simulink model "Bio_Digital_Twin"  (R2025b)
settings: Solver=VariableStepAuto  StartTime=0.0  StopTime=10.0  RelTol=1e-3
undefined symbols (not defined in the file): dspblkCoreblockFVToolHelper, gcbh
libraries: simulink x15, dspstat3 x4
(part 2 of 2)

== system Bio_Digital_Twin/Frugal_AI/4.5_Risk_Fusion_Decision_logic ==
  In1 : Inport  OutDataTypeStr=double
  SPO2_Mean : Inport  Port=2  OutDataTypeStr=double
  HR_Mean : Inport  Port=3  OutDataTypeStr=double
  In2 : Inport  Port=4  OutDataTypeStr=double
  Global_Health_State : Inport  Port=5  OutDataTypeStr=double
  Temp_Mean : Inport  Port=6  OutDataTypeStr=double
  In4 : Inport  Port=7  OutDataTypeStr=double
  HR_Flag : Inport  Port=8  OutDataTypeStr=double
  SPO2_Flag : Inport  Port=9  OutDataTypeStr=double
  TEMP_Flag : Inport  Port=10  OutDataTypeStr=double
  4.5.1_Risk_Signal_Normalizer : Subsystem
      settings: PortSchema="{\"entries\":[{\"content\":{\"sides\":[{\"content\":{},\"type\":\"ConnectorPlacement.EquallySpacedRectSide\",\"uuid\":\"8f35f634-c66e-422d-9c58-c61a4ee3cb54\"},{\"content\":{\"connectorIds\":[\"Out1\",\"Out2\",\"Out3\"],\"side\":\"RIGHT\"},\"type\":\"ConnectorPlacement.EquallySpacedRectSide\",\"uuid\":\"9f9283e6-4c64-451c-ad49-820c1276ee73\"},{\"content\":{\"side\":\"TOP\"},\"type\":\"ConnectorPlacement.EquallySpacedRectSide\",\"uuid\":\"18598fd6-31f1-4989-a958-abe44ef931de\"},{\"content\":{\"connectorIds\":[\"In1\",\"In2\",\"In3\"],\"side\":\"BOTTOM\"},\"type\":\"ConnectorPlacement.EquallySpacedRectSide\",\"uuid\":\"37672f05-fc1d-406b-b410-c6708a58aa07\"}]},\"type\":\"ConnectorPlacement.EquallySpacedConnector\",\"uuid\":\"a95a04c5-95c4-48ce-b08e-1a83caf92d36\"}],\"packageUris\":[\"http://schema.mathworks.com/mf0/Connector/R2020b\"],\"version\":\"1.0\"}"
  4.5.2_Physiological_Context_Moniter : Subsystem
      settings: PortSchema="{\"entries\":[{\"content\":{\"sides\":[{\"content\":{},\"type\":\"ConnectorPlacement.EquallySpacedRectSide\",\"uuid\":\"ba542400-0cd1-4e31-b99c-7003472743bf\"},{\"content\":{\"connectorIds\":[\"Out1\",\"Out2\",\"Out3\"],\"side\":\"RIGHT\"},\"type\":\"ConnectorPlacement.EquallySpacedRectSide\",\"uuid\":\"eb7b6bce-55bf-4921-bc52-6edeb25fab9e\"},{\"content\":{\"connectorIds\":[\"In1\",\"In2\",\"In3\"],\"side\":\"TOP\"},\"type\":\"ConnectorPlacement.EquallySpacedRectSide\",\"uuid\":\"71120ea0-ac95-49d2-9d4b-92656524cc31\"}]},\"type\":\"ConnectorPlacement.EquallySpacedConnector\",\"uuid\":\"9e07e074-34e6-4f09-a71b-3d251b7224e4\"}],\"packageUris\":[\"http://schema.mathworks.com/mf0/Connector/R2020b\"],\"version\":\"1.0\"}"
  4.5.3_Weighted_Risk_Fusion_Core : Subsystem
      settings: PortSchema="{\"entries\":[{\"content\":{\"sides\":[{\"content\":{\"connectorIds\":[\"In1\",\"In2\",\"In3\"]},\"type\":\"ConnectorPlacement.EquallySpacedRectSide\",\"uuid\":\"8f35f634-c66e-422d-9c58-c61a4ee3cb54\"},{\"content\":{\"connectorIds\":[\"Out1\"],\"side\":\"RIGHT\"},\"type\":\"ConnectorPlacement.EquallySpacedRectSide\",\"uuid\":\"9f9283e6-4c64-451c-ad49-820c1276ee73\"},{\"content\":{\"connectorIds\":[\"In4\",\"In5\",\"In6\"],\"side\":\"TOP\"},\"type\":\"ConnectorPlacement.EquallySpacedRectSide\",\"uuid\":\"18598fd6-31f1-4989-a958-abe44ef931de\"}]},\"type\":\"ConnectorPlacement.EquallySpacedConnector\",\"uuid\":\"a95a04c5-95c4-48ce-b08e-1a83caf92d36\"}],\"packageUris\":[\"http://schema.mathworks.com/mf0/Connector/R2020b\"],\"version\":\"1.0\"}"
  4.5.4_Discrete_Override_Logic : Subsystem
      settings: PortSchema="{\"entries\":[{\"content\":{\"sides\":[{\"content\":{},\"type\":\"ConnectorPlacement.EquallySpacedRectSide\",\"uuid\":\"ba542400-0cd1-4e31-b99c-7003472743bf\"},{\"content\":{\"connectorIds\":[\"Out1\",\"Out2\"],\"side\":\"RIGHT\"},\"type\":\"ConnectorPlacement.EquallySpacedRectSide\",\"uuid\":\"eb7b6bce-55bf-4921-bc52-6edeb25fab9e\"},{\"content\":{\"connectorIds\":[\"In1\"],\"side\":\"TOP\"},\"type\":\"ConnectorPlacement.EquallySpacedRectSide\",\"uuid\":\"71120ea0-ac95-49d2-9d4b-92656524cc31\"},{\"content\":{\"connectorIds\":[\"In2\",\"In3\",\"In4\",\"In5\"],\"side\":\"BOTTOM\"},\"type\":\"ConnectorPlacement.EquallySpacedRectSide\",\"uuid\":\"ed423af9-15f8-4a33-aaec-371b081b1cbe\"}]},\"type\":\"ConnectorPlacement.EquallySpacedConnector\",\"uuid\":\"9e07e074-34e6-4f09-a71b-3d251b7224e4\"}],\"packageUris\":[\"http://schema.mathworks.com/mf0/Connector/R2020b\"],\"version\":\"1.0\"}"
  4.5.5_Final_Risk_Selecter&Decision_Output : Subsystem
      settings: PortSchema="{\"entries\":[{\"content\":{\"sides\":[{\"content\":{\"connectorIds\":[\"In1\",\"In2\"]},\"type\":\"ConnectorPlacement.EquallySpacedRectSide\",\"uuid\":\"1398e62b-675a-459d-b341-3a2d58b0042e\"},{\"content\":{\"connectorIds\":[\"Out1\",\"Out2\",\"Out3\",\"Out4\"],\"side\":\"RIGHT\"},\"type\":\"ConnectorPlacement.EquallySpacedRectSide\",\"uuid\":\"49b971ab-5b3e-431b-b022-6e647649d68a\"},{\"content\":{\"connectorIds\":[\"In3\",\"Out5\"],\"side\":\"TOP\"},\"type\":\"ConnectorPlacement.EquallySpacedRectSide\",\"uuid\":\"481e4b75-ca94-4b8e-ac5a-54646a036782\"}]},\"type\":\"ConnectorPlacement.EquallySpacedConnector\",\"uuid\":\"3a2d46a4-3de7-4d3b-b474-f54ea7c5581f\"}],\"packageUris\":[\"http://schema.mathworks.com/mf0/Connector/R2020b\"],\"version\":\"1.0\"}"
  Scope : Scope
      settings: DataLoggingVariableName=ScopeData76  DataLoggingSaveFormat=Array
  Scope1 : Scope
      settings: DataLoggingVariableName=ScopeData77  DataLoggingSaveFormat=Array
  Risk_Level : Outport
  Global_Risk_Index : Outport  Port=2
  Over_Ride_Flag : Outport  Port=3
  wires:
  In1/1 -> 4.5.1_Risk_Signal_Normalizer/1(HR_Risk_Score)
  In2/1 -> 4.5.1_Risk_Signal_Normalizer/3(SPO2_Risk_Score)
  In4/1 -> 4.5.1_Risk_Signal_Normalizer/2(TEMP_Risk_Score)
  HR_Mean/1 -> 4.5.2_Physiological_Context_Moniter/1(HR_Mean)
  SPO2_Mean/1 -> 4.5.2_Physiological_Context_Moniter/2(SPO2_Mean)
  Temp_Mean/1 -> 4.5.2_Physiological_Context_Moniter/3(Temp_Mean)
  4.5.2_Physiological_Context_Moniter/1(HR_Context_Risk) -> 4.5.3_Weighted_Risk_Fusion_Core/6(HR_Context_Risk)
  4.5.2_Physiological_Context_Moniter/2(TEMP_Context_Risk) -> 4.5.3_Weighted_Risk_Fusion_Core/3(TEMP_Context_Risk)
  4.5.2_Physiological_Context_Moniter/3(SPO2_Context_Risk) -> 4.5.3_Weighted_Risk_Fusion_Core/1(SPO2_Context_Risk)
  Global_Health_State/1 -> 4.5.4_Discrete_Override_Logic/2(Global_Health_State)
  4.5.3_Weighted_Risk_Fusion_Core/1(Global_Risk_Index) -> 4.5.5_Final_Risk_Selecter&Decision_Output/3(Global_Risk_Index), 4.5.4_Discrete_Override_Logic/1(Global_Risk_Index)
  HR_Flag/1 -> 4.5.4_Discrete_Override_Logic/3(HR_Flag)
  SPO2_Flag/1 -> 4.5.4_Discrete_Override_Logic/5(SPO2_Flag)
  TEMP_Flag/1 -> 4.5.4_Discrete_Override_Logic/4(TEMP_Flag)
  4.5.1_Risk_Signal_Normalizer/1(HR_Risk_Norm) -> 4.5.3_Weighted_Risk_Fusion_Core/5(HR_Risk_Norm)
  4.5.1_Risk_Signal_Normalizer/2(SPO2_Risk_Norm) -> 4.5.3_Weighted_Risk_Fusion_Core/4(SPO2_Risk_Norm)
  4.5.1_Risk_Signal_Normalizer/3(TEMP_Risk_Norm) -> 4.5.3_Weighted_Risk_Fusion_Core/2(TEMP_Risk_Norm)
  4.5.4_Discrete_Override_Logic/1(Override_level) -> 4.5.5_Final_Risk_Selecter&Decision_Output/2(Override_level)
  4.5.4_Discrete_Override_Logic/2(Out1) -> 4.5.5_Final_Risk_Selecter&Decision_Output/1(Override_Flag)
  4.5.5_Final_Risk_Selecter&Decision_Output/1(Out1) -> Scope/1
  4.5.5_Final_Risk_Selecter&Decision_Output/2(Out2) -> Scope1/1
  4.5.5_Final_Risk_Selecter&Decision_Output/5(Out3) -> Global_Risk_Index/1
  4.5.5_Final_Risk_Selecter&Decision_Output/3(Out4) -> Risk_Level/1
  4.5.5_Final_Risk_Selecter&Decision_Output/4(Out5) -> Over_Ride_Flag/1

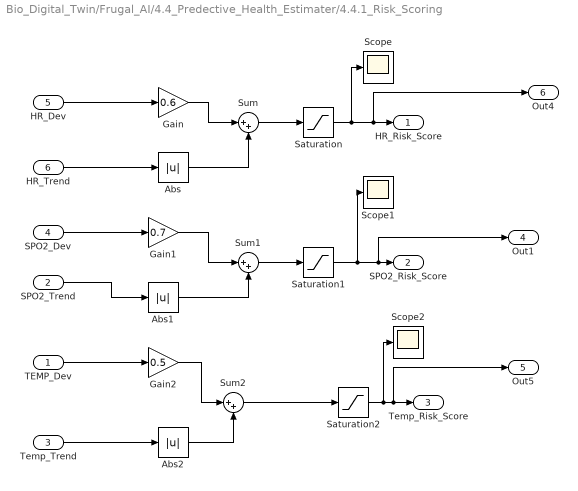
== system Bio_Digital_Twin/Frugal_AI/4.4_Predective_Health_Estimater/4.4.1_Risk_Scoring ==
  TEMP_Dev : Inport
  SPO2_Trend : Inport  Port=2
  Temp_Trend : Inport  Port=3
  SPO2_Dev : Inport  Port=4
  HR_Dev : Inport  Port=5  OutDataTypeStr=double
  HR_Trend : Inport  Port=6
  Abs : Abs  ZeroCross=off  OutDataTypeStr=double  SaturateOnIntegerOverflow=off
  Abs1 : Abs  ZeroCross=off  SaturateOnIntegerOverflow=off
  Abs2 : Abs  ZeroCross=off  SaturateOnIntegerOverflow=off
  Gain : Gain  Gain=0.6
  Gain1 : Gain  Gain=0.7
  Gain2 : Gain  Gain=0.5
  Saturation : Saturate  UpperLimit=1  LowerLimit=0  ZeroCross=off
  Saturation1 : Saturate  UpperLimit=1  LowerLimit=0  ZeroCross=off
  Saturation2 : Saturate  UpperLimit=1  LowerLimit=0  ZeroCross=off
  Scope : Scope
      settings: DataLoggingVariableName=ScopeData38  DataLoggingSaveFormat=Array
  Scope1 : Scope
      settings: ActiveDisplayYMinimum=-0.029651653403424238  ActiveDisplayYMaximum=1.5657002997215752  DataLoggingVariableName=ScopeData39  DataLoggingSaveFormat=Array
  Scope2 : Scope
      settings: DataLoggingVariableName=ScopeData40  DataLoggingSaveFormat=Array
  Sum : Sum  Inputs=|++
  Sum1 : Sum  Inputs=|++
  Sum2 : Sum  Inputs=|++
  HR_Risk_Score : Outport  VectorParamsAs1DForOutWhenUnconnected=off
  SPO2_Risk_Score : Outport  Port=2  VectorParamsAs1DForOutWhenUnconnected=off
  Temp_Risk_Score : Outport  Port=3  VectorParamsAs1DForOutWhenUnconnected=off
  Out1 : Outport  Port=4
  Out5 : Outport  Port=5
  Out4 : Outport  Port=6
  wires:
  HR_Trend/1 -> Abs/1
  HR_Dev/1 -> Gain/1
  Gain/1 -> Sum/1
  Abs/1 -> Sum/2
  Sum/1 -> Saturation/1
  Saturation/1 -> Scope/1, Out4/1, HR_Risk_Score/1
  SPO2_Dev/1 -> Gain1/1
  SPO2_Trend/1 -> Abs1/1
  Gain1/1 -> Sum1/1
  Abs1/1 -> Sum1/2
  Sum1/1 -> Saturation1/1
  Saturation1/1 -> Scope1/1, Out1/1, SPO2_Risk_Score/1
  TEMP_Dev/1 -> Gain2/1
  Temp_Trend/1 -> Abs2/1
  Gain2/1 -> Sum2/1
  Abs2/1 -> Sum2/2
  Sum2/1 -> Saturation2/1
  Saturation2/1 -> Scope2/1, Out5/1, Temp_Risk_Score/1

== system Bio_Digital_Twin/Frugal_AI/4.4_Predective_Health_Estimater/4.4.2_Trend_Penetration ==
  HR_Trend : Inport
  SPO2_Trend : Inport  Port=2
  Temp_Trend : Inport  Port=3
  Abs : Abs  ZeroCross=off  SaturateOnIntegerOverflow=off
  Abs1 : Abs  ZeroCross=off  SaturateOnIntegerOverflow=off
  Abs2 : Abs  ZeroCross=off  SaturateOnIntegerOverflow=off
  Gain : Gain  Gain=0.3
  Gain1 : Gain  Gain=0.6
  Gain2 : Gain  Gain=1.2
  Saturation : Saturate  UpperLimit=0.3  LowerLimit=0  ZeroCross=off
  Saturation1 : Saturate  UpperLimit=0.20  LowerLimit=0  ZeroCross=off
  Saturation2 : Saturate  UpperLimit=0.25  LowerLimit=0  ZeroCross=off
  Scope : Scope
      settings: ActiveDisplayYMinimum=-0.037499999999999992  ActiveDisplayYMaximum=0.33749999999999997  DataLoggingVariableName=ScopeData41  DataLoggingSaveFormat=Array
  Scope1 : Scope
      settings: ActiveDisplayYMinimum=-0.024999999999999994  ActiveDisplayYMaximum=0.225  DataLoggingVariableName=ScopeData42  DataLoggingSaveFormat=Array
  Scope2 : Scope
      settings: ActiveDisplayYMinimum=-0.031249999999999993  ActiveDisplayYMaximum=0.28125  DataLoggingVariableName=ScopeData43  DataLoggingSaveFormat=Array
  HR_Trend_Penalty : Outport
  SPO2_Trend_Penality : Outport  Port=2
  TEMP_Penality : Outport  Port=3
  wires:
  HR_Trend/1 -> Abs/1
  Saturation/1 -> Scope/1, HR_Trend_Penalty/1
  Gain/1 -> Saturation/1
  Abs/1 -> Gain/1
  SPO2_Trend/1 -> Abs1/1
  Temp_Trend/1 -> Abs2/1
  Abs2/1 -> Gain2/1
  Gain2/1 -> Saturation2/1
  Saturation2/1 -> Scope2/1, TEMP_Penality/1
  Abs1/1 -> Gain1/1
  Gain1/1 -> Saturation1/1
  Saturation1/1 -> Scope1/1, SPO2_Trend_Penality/1

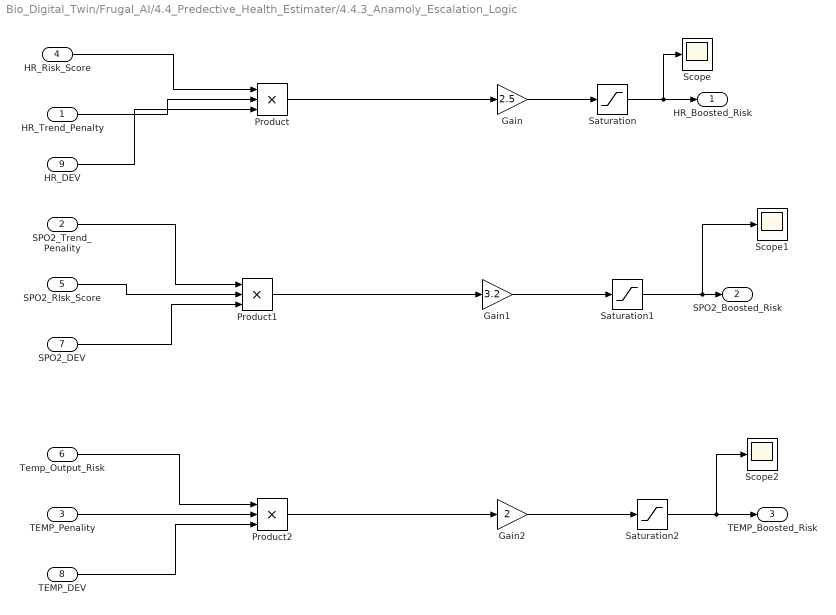
== system Bio_Digital_Twin/Frugal_AI/4.4_Predective_Health_Estimater/4.4.3_Anamoly_Escalation_Logic ==
  HR_Trend_Penalty : Inport
  SPO2_Trend_Penality : Inport  Port=2
  TEMP_Penality : Inport  Port=3
  HR_Risk_Score : Inport  Port=4
  SPO2_RIsk_Score : Inport  Port=5
  Temp_Output_Risk : Inport  Port=6
  SPO2_DEV : Inport  Port=7
  TEMP_DEV : Inport  Port=8
  HR_DEV : Inport  Port=9
  Gain : Gain  Gain=2.5
  Gain1 : Gain  Gain=3.2
  Gain2 : Gain  Gain=2
  Product : Product  Inputs=3
  Product1 : Product  Inputs=3
  Product2 : Product  Inputs=3
  Saturation : Saturate  UpperLimit=1  LowerLimit=0  ZeroCross=off
  Saturation1 : Saturate  UpperLimit=1  LowerLimit=0  ZeroCross=off
  Saturation2 : Saturate  UpperLimit=1  LowerLimit=0  ZeroCross=off
  Scope : Scope
      settings: ActiveDisplayYMinimum=-0.076388475038902851  ActiveDisplayYMaximum=0.68749627535012581  DataLoggingVariableName=ScopeData44  DataLoggingSaveFormat=Array
  Scope1 : Scope
      settings: ActiveDisplayYMinimum=-0.067702104531752558  ActiveDisplayYMaximum=0.60931894078577309  DataLoggingVariableName=ScopeData45  DataLoggingSaveFormat=Array
  Scope2 : Scope
      settings: ActiveDisplayYMinimum=-0.0094894903527777043  ActiveDisplayYMaximum=0.085405413174999362  DataLoggingVariableName=ScopeData46  DataLoggingSaveFormat=Array
  HR_Boosted_Risk : Outport  VectorParamsAs1DForOutWhenUnconnected=off
  SPO2_Boosted_Risk : Outport  Port=2
  TEMP_Boosted_Risk : Outport  Port=3
  wires:
  HR_Risk_Score/1 -> Product/1
  HR_Trend_Penalty/1 -> Product/2
  HR_DEV/1 -> Product/3
  SPO2_Trend_Penality/1 -> Product1/1
  SPO2_RIsk_Score/1 -> Product1/2
  SPO2_DEV/1 -> Product1/3
  Temp_Output_Risk/1 -> Product2/1
  TEMP_Penality/1 -> Product2/2
  TEMP_DEV/1 -> Product2/3
  Product/1 -> Gain/1
  Gain/1 -> Saturation/1
  Saturation/1 -> Scope/1, HR_Boosted_Risk/1
  Gain2/1 -> Saturation2/1
  Gain1/1 -> Saturation1/1
  Saturation1/1 -> Scope1/1, SPO2_Boosted_Risk/1
  Saturation2/1 -> Scope2/1, TEMP_Boosted_Risk/1
  Product1/1 -> Gain1/1
  Product2/1 -> Gain2/1

== system Bio_Digital_Twin/Frugal_AI/4.4_Predective_Health_Estimater/4.4.4_Vital_Fusion_Engine ==
  SPO2_Trend_Penality : Inport
  TEMP_Boosted_Risk : Inport  Port=2
  HR_Boosted_Risk : Inport  Port=3
  TEMP_Trend_Penality : Inport  Port=4
  TEMP_Flag : Inport  Port=5
  HR_Trend_Penalty : Inport  Port=6
  HR_Flag : Inport  Port=7
  SPO2_Flag : Inport  Port=8
  SPO2_Boosted_Risk : Inport  Port=9
  4.4.4.1_Weighted_Risk_Aggregator : Subsystem
      settings: PortSchema="{\"entries\":[{\"content\":{\"sides\":[{\"content\":{},\"type\":\"ConnectorPlacement.EquallySpacedRectSide\",\"uuid\":\"737bb885-e7c9-4573-85e5-b83dda6485f1\"},{\"content\":{\"connectorIds\":[\"Out1\"],\"side\":\"RIGHT\"},\"type\":\"ConnectorPlacement.EquallySpacedRectSide\",\"uuid\":\"740a03a9-133d-4f41-bb19-7b5e8b3a8d7e\"},{\"content\":{\"connectorIds\":[\"In1\"],\"side\":\"TOP\"},\"type\":\"ConnectorPlacement.EquallySpacedRectSide\",\"uuid\":\"4008c6be-6fbc-4f8a-ab91-2e671a35a61f\"},{\"content\":{\"connectorIds\":[\"In2\",\"In3\"],\"side\":\"BOTTOM\"},\"type\":\"ConnectorPlacement.EquallySpacedRectSide\",\"uuid\":\"541123af-325e-4018-abd6-217c806ff677\"}]},\"type\":\"ConnectorPlacement.EquallySpacedConnector\",\"uuid\":\"4bffb07e-74c2-4f1f-82f1-4306adc281b9\"}],\"packageUris\":[\"http://schema.mathworks.com/mf0/Connector/R2020b\"],\"version\":\"1.0\"}"
  4.4.4.2_Trend_Reinforcement_Logic : Subsystem
      settings: PortSchema="{\"entries\":[{\"content\":{\"sides\":[{\"content\":{},\"type\":\"ConnectorPlacement.EquallySpacedRectSide\",\"uuid\":\"25541af2-9525-4f8c-abbb-22df26048cee\"},{\"content\":{\"connectorIds\":[\"Out1\"],\"side\":\"RIGHT\"},\"type\":\"ConnectorPlacement.EquallySpacedRectSide\",\"uuid\":\"1363b628-3ee9-451f-9ff9-7a32b3bff014\"},{\"content\":{\"side\":\"TOP\"},\"type\":\"ConnectorPlacement.EquallySpacedRectSide\",\"uuid\":\"085c579b-f7a8-4980-bc39-19f414c4d171\"},{\"content\":{\"connectorIds\":[\"In1\",\"In2\",\"In3\"],\"side\":\"BOTTOM\"},\"type\":\"ConnectorPlacement.EquallySpacedRectSide\",\"uuid\":\"8648316c-16bf-41e8-ae35-abe9e87cf577\"}]},\"type\":\"ConnectorPlacement.EquallySpacedConnector\",\"uuid\":\"fb659e6d-00b5-4060-933b-4a03338751c4\"}],\"packageUris\":[\"http://schema.mathworks.com/mf0/Connector/R2020b\"],\"version\":\"1.0\"}"
  4.4.4.3_Flag_Confidence_Gate : Subsystem
      settings: PortSchema="{\"entries\":[{\"content\":{\"sides\":[{\"content\":{},\"type\":\"ConnectorPlacement.EquallySpacedRectSide\",\"uuid\":\"25541af2-9525-4f8c-abbb-22df26048cee\"},{\"content\":{\"connectorIds\":[\"Out1\"],\"side\":\"RIGHT\"},\"type\":\"ConnectorPlacement.EquallySpacedRectSide\",\"uuid\":\"1363b628-3ee9-451f-9ff9-7a32b3bff014\"},{\"content\":{\"connectorIds\":[\"In1\"],\"side\":\"TOP\"},\"type\":\"ConnectorPlacement.EquallySpacedRectSide\",\"uuid\":\"085c579b-f7a8-4980-bc39-19f414c4d171\"},{\"content\":{\"connectorIds\":[\"In2\",\"In3\",\"In4\"],\"side\":\"BOTTOM\"},\"type\":\"ConnectorPlacement.EquallySpacedRectSide\",\"uuid\":\"37001957-af6f-4dd2-a4d8-c32bc34d5802\"}]},\"type\":\"ConnectorPlacement.EquallySpacedConnector\",\"uuid\":\"fb659e6d-00b5-4060-933b-4a03338751c4\"}],\"packageUris\":[\"http://schema.mathworks.com/mf0/Connector/R2020b\"],\"version\":\"1.0\"}"
  4.4.4.4_Final_risk_Normalizer : Subsystem
  4.4.4.5_Decision&Drug_Trigger_Logic : Subsystem
      settings: PortSchema="{\"entries\":[{\"content\":{\"sides\":[{\"content\":{},\"type\":\"ConnectorPlacement.EquallySpacedRectSide\",\"uuid\":\"737bb885-e7c9-4573-85e5-b83dda6485f1\"},{\"content\":{\"connectorIds\":[\"Out1\"],\"side\":\"RIGHT\"},\"type\":\"ConnectorPlacement.EquallySpacedRectSide\",\"uuid\":\"740a03a9-133d-4f41-bb19-7b5e8b3a8d7e\"},{\"content\":{\"connectorIds\":[\"In1\"],\"side\":\"TOP\"},\"type\":\"ConnectorPlacement.EquallySpacedRectSide\",\"uuid\":\"4008c6be-6fbc-4f8a-ab91-2e671a35a61f\"}]},\"type\":\"ConnectorPlacement.EquallySpacedConnector\",\"uuid\":\"4bffb07e-74c2-4f1f-82f1-4306adc281b9\"}],\"packageUris\":[\"http://schema.mathworks.com/mf0/Connector/R2020b\"],\"version\":\"1.0\"}"
  wires:
  HR_Boosted_Risk/1 -> 4.4.4.1_Weighted_Risk_Aggregator/3(HR_Boosted_Risk)
  SPO2_Boosted_Risk/1 -> 4.4.4.1_Weighted_Risk_Aggregator/2(SPO2_Boosted_Risk)
  TEMP_Boosted_Risk/1 -> 4.4.4.1_Weighted_Risk_Aggregator/1(TEMP_Boosted_Risk)
  SPO2_Trend_Penality/1 -> 4.4.4.2_Trend_Reinforcement_Logic/1(SPO2_Trend_Penality)
  HR_Trend_Penalty/1 -> 4.4.4.2_Trend_Reinforcement_Logic/2(HR_Trend_Penalty)
  TEMP_Trend_Penality/1 -> 4.4.4.2_Trend_Reinforcement_Logic/3(TEMP_Trend_Penality)
  HR_Flag/1 -> 4.4.4.3_Flag_Confidence_Gate/2(HR_Flag)
  SPO2_Flag/1 -> 4.4.4.3_Flag_Confidence_Gate/4(SPO2_Flag)
  TEMP_Flag/1 -> 4.4.4.3_Flag_Confidence_Gate/3(TEMP_Flag)
  4.4.4.2_Trend_Reinforcement_Logic/1(Trend_Factor) -> 4.4.4.4_Final_risk_Normalizer/3(Trend_Factor), 4.4.4.3_Flag_Confidence_Gate/1(Trend_Factor)
  4.4.4.1_Weighted_Risk_Aggregator/1(R_Weighted) -> 4.4.4.4_Final_risk_Normalizer/1(R_Weighted)
  4.4.4.3_Flag_Confidence_Gate/1(Risk_Validated) -> 4.4.4.4_Final_risk_Normalizer/2(Risk_Validated)
  4.4.4.4_Final_risk_Normalizer/1(Vital_Risk_Score) -> 4.4.4.5_Decision&Drug_Trigger_Logic/1(Vital_Risk_Score)

== system Bio_Digital_Twin/Frugal_AI/4.4_Predective_Health_Estimater/4.4.5_Health_State_Encoder ==
  HR_Risk_Score : Inport  OutDataTypeStr=double
  SPO2_RIsk_Score : Inport  Port=2  OutDataTypeStr=double
  Temp_Risk_Output : Inport  Port=3  OutDataTypeStr=double
  TEMP_Flag : Inport  Port=4  OutDataTypeStr=double
  HR_Flag : Inport  Port=5
  SPO2_Flag : Inport  Port=6  OutDataTypeStr=double
  4.4.5.1_Vital_Severity_Normalizer : Subsystem
      settings: PortSchema="{\"entries\":[{\"content\":{\"sides\":[{\"content\":{\"connectorIds\":[\"In1\"]},\"type\":\"ConnectorPlacement.EquallySpacedRectSide\",\"uuid\":\"25541af2-9525-4f8c-abbb-22df26048cee\"},{\"content\":{\"connectorIds\":[\"In6\",\"Out1\",\"Out2\",\"Out3\"],\"side\":\"RIGHT\"},\"type\":\"ConnectorPlacement.EquallySpacedRectSide\",\"uuid\":\"1363b628-3ee9-451f-9ff9-7a32b3bff014\"},{\"content\":{\"side\":\"TOP\"},\"type\":\"ConnectorPlacement.EquallySpacedRectSide\",\"uuid\":\"085c579b-f7a8-4980-bc39-19f414c4d171\"},{\"content\":{\"connectorIds\":[\"In2\",\"In3\",\"In4\",\"In5\"],\"side\":\"BOTTOM\"},\"type\":\"ConnectorPlacement.EquallySpacedRectSide\",\"uuid\":\"3b4b4325-d39e-4c80-9f50-c26047788f8b\"}]},\"type\":\"ConnectorPlacement.EquallySpacedConnector\",\"uuid\":\"fb659e6d-00b5-4060-933b-4a03338751c4\"}],\"packageUris\":[\"http://schema.mathworks.com/mf0/Connector/R2020b\"],\"version\":\"1.0\"}"
  4.4.5.2_Health_Vector_Builder : Subsystem
  4.4.5.3_Weighted_Health_Index_generator : Subsystem
  4.4.5.4_Discrete_Health_State_Classifier : Subsystem
  4.4.5.5_Final_Decision : Subsystem
      settings: PortSchema="{\"entries\":[{\"content\":{\"sides\":[{\"content\":{\"connectorIds\":[\"In1\"]},\"type\":\"ConnectorPlacement.EquallySpacedRectSide\",\"uuid\":\"25541af2-9525-4f8c-abbb-22df26048cee\"},{\"content\":{\"connectorIds\":[\"Out1\"],\"side\":\"RIGHT\"},\"type\":\"ConnectorPlacement.EquallySpacedRectSide\",\"uuid\":\"1363b628-3ee9-451f-9ff9-7a32b3bff014\"},{\"content\":{\"connectorIds\":[\"In2\",\"In3\"],\"side\":\"TOP\"},\"type\":\"ConnectorPlacement.EquallySpacedRectSide\",\"uuid\":\"085c579b-f7a8-4980-bc39-19f414c4d171\"},{\"content\":{\"connectorIds\":[\"In4\"],\"side\":\"BOTTOM\"},\"type\":\"ConnectorPlacement.EquallySpacedRectSide\",\"uuid\":\"6701486d-dcdb-4b0d-ba3b-9fb711ea3ea4\"}]},\"type\":\"ConnectorPlacement.EquallySpacedConnector\",\"uuid\":\"fb659e6d-00b5-4060-933b-4a03338751c4\"}],\"packageUris\":[\"http://schema.mathworks.com/mf0/Connector/R2020b\"],\"version\":\"1.0\"}"
  Global_Health_State : Outport  OutDataTypeStr=double  VectorParamsAs1DForOutWhenUnconnected=off
  wires:
  TEMP_Flag/1 -> 4.4.5.1_Vital_Severity_Normalizer/1(TEMP_Flag)
  SPO2_Flag/1 -> 4.4.5.1_Vital_Severity_Normalizer/5(SPO2_Flag)
  HR_Flag/1 -> 4.4.5.1_Vital_Severity_Normalizer/6(HR_Flag)
  4.4.5.1_Vital_Severity_Normalizer/1(HR_Severity) -> 4.4.5.2_Health_Vector_Builder/1(HR_Severity)
  4.4.5.1_Vital_Severity_Normalizer/2(SPO2_Severity) -> 4.4.5.2_Health_Vector_Builder/2(SPO2_Severity)
  4.4.5.1_Vital_Severity_Normalizer/3(TEMP_Severity) -> 4.4.5.2_Health_Vector_Builder/3(TEMP_Severity)
  4.4.5.2_Health_Vector_Builder/1(Health_Vector) -> 4.4.5.3_Weighted_Health_Index_generator/1(Health_Vector)
  4.4.5.2_Health_Vector_Builder/2(Out1) -> 4.4.5.4_Discrete_Health_State_Classifier/1(HR_Severity)
  4.4.5.2_Health_Vector_Builder/3(Out2) -> 4.4.5.4_Discrete_Health_State_Classifier/2(SPO2_Severity)
  4.4.5.4_Discrete_Health_State_Classifier/1(HR_Health_State) -> 4.4.5.5_Final_Decision/2(HR_Health_State)
  4.4.5.4_Discrete_Health_State_Classifier/2(SPO2_Health_state) -> 4.4.5.5_Final_Decision/3(SPO2_Health_state)
  4.4.5.4_Discrete_Health_State_Classifier/3(TEMP_Health_State) -> 4.4.5.5_Final_Decision/4(TEMP_Health_State)
  4.4.5.2_Health_Vector_Builder/4(Out3) -> 4.4.5.4_Discrete_Health_State_Classifier/3(TEMP_Severity)
  HR_Risk_Score/1 -> 4.4.5.1_Vital_Severity_Normalizer/2(HR_Risk_Score)
  SPO2_RIsk_Score/1 -> 4.4.5.1_Vital_Severity_Normalizer/4(SPO2_RIsk_Score)
  Temp_Risk_Output/1 -> 4.4.5.1_Vital_Severity_Normalizer/3(Temp_Risk_Output)
  4.4.5.3_Weighted_Health_Index_generator/1(Health_Index) -> 4.4.5.5_Final_Decision/1(Health_Index)
  4.4.5.5_Final_Decision/1(Global_Health_State) -> Global_Health_State/1

== system Bio_Digital_Twin/Frugal_AI/4.5_Risk_Fusion_Decision_logic/4.5.1_Risk_Signal_Normalizer ==
  HR_Risk_Score : Inport  OutDataTypeStr=double
  TEMP_Risk_Score : Inport  Port=2  OutDataTypeStr=double
  SPO2_Risk_Score : Inport  Port=3  OutDataTypeStr=double
  Saturation : Saturate  UpperLimit=1  LowerLimit=0  ZeroCross=off  OutDataTypeStr=double
  Saturation1 : Saturate  UpperLimit=1  LowerLimit=0  ZeroCross=off  OutDataTypeStr=double
  Saturation2 : Saturate  UpperLimit=1  LowerLimit=0  ZeroCross=off  OutDataTypeStr=double
  Scope : Scope
      settings: DataLoggingVariableName=ScopeData64  DataLoggingSaveFormat=Array
  Scope1 : Scope
      settings: DataLoggingVariableName=ScopeData65  DataLoggingSaveFormat=Array
  Scope2 : Scope
      settings: DataLoggingVariableName=ScopeData66  DataLoggingSaveFormat=Array
  HR_Risk_Norm : Outport  OutDataTypeStr=double
  SPO2_Risk_Norm : Outport  Port=2  OutDataTypeStr=double
  TEMP_Risk_Norm : Outport  Port=3  OutDataTypeStr=double
  wires:
  HR_Risk_Score/1 -> Saturation/1
  Saturation/1 -> Scope/1, HR_Risk_Norm/1
  SPO2_Risk_Score/1 -> Saturation2/1
  TEMP_Risk_Score/1 -> Saturation1/1
  Saturation2/1 -> Scope2/1, SPO2_Risk_Norm/1
  Saturation1/1 -> TEMP_Risk_Norm/1, Scope1/1

== system Bio_Digital_Twin/Frugal_AI/4.5_Risk_Fusion_Decision_logic/4.5.2_Physiological_Context_Moniter ==
  HR_Mean : Inport  OutDataTypeStr=double
  SPO2_Mean : Inport  Port=2  OutDataTypeStr=double
  Temp_Mean : Inport  Port=3  OutDataTypeStr=double
  Gain : Gain  Gain=1/100  OutDataTypeStr=double
  Gain1 : Gain  Gain=1/100  OutDataTypeStr=double
  Gain2 : Gain  Gain=1/50  OutDataTypeStr=double
  Scope : Scope
      settings: DataLoggingVariableName=ScopeData68  DataLoggingSaveFormat=Array
  Scope1 : Scope
      settings: DataLoggingVariableName=ScopeData69  DataLoggingSaveFormat=Array
  Scope2 : Scope
      settings: DataLoggingVariableName=ScopeData70  DataLoggingSaveFormat=Array
  HR_Context_Risk : Outport  OutDataTypeStr=double
  TEMP_Context_Risk : Outport  Port=2  OutDataTypeStr=double
  SPO2_Context_Risk : Outport  Port=3  OutDataTypeStr=double
  wires:
  HR_Mean/1 -> Gain/1
  Temp_Mean/1 -> Gain2/1
  SPO2_Mean/1 -> Gain1/1
  Gain/1 -> Scope/1, HR_Context_Risk/1
  Gain2/1 -> Scope2/1, TEMP_Context_Risk/1
  Gain1/1 -> Scope1/1, SPO2_Context_Risk/1

== system Bio_Digital_Twin/Frugal_AI/4.5_Risk_Fusion_Decision_logic/4.5.3_Weighted_Risk_Fusion_Core ==
  SPO2_Context_Risk : Inport  OutDataTypeStr=double
  TEMP_Risk_Norm : Inport  Port=2  OutDataTypeStr=double
  TEMP_Context_Risk : Inport  Port=3  OutDataTypeStr=double
  SPO2_Risk_Norm : Inport  Port=4  OutDataTypeStr=double
  HR_Risk_Norm : Inport  Port=5  OutDataTypeStr=double
  HR_Context_Risk : Inport  Port=6  OutDataTypeStr=double
  Gain : Gain  Gain=0.4  OutDataTypeStr=double
  Gain1 : Gain  Gain=0.4  OutDataTypeStr=double
  Gain2 : Gain  Gain=0.4  OutDataTypeStr=double
  Gain3 : Gain  OutDataTypeStr=double
  Gain4 : Gain  OutDataTypeStr=double
  Gain5 : Gain  OutDataTypeStr=double
  Saturation : Saturate  UpperLimit=1  LowerLimit=0  ZeroCross=off  OutDataTypeStr=double
  Scope : Scope
      settings: DataLoggingVariableName=ScopeData71  DataLoggingSaveFormat=Array
  Sum : Sum  Inputs=|++++++  OutDataTypeStr=double
  Global_Risk_Index : Outport  OutDataTypeStr=double
  wires:
  HR_Context_Risk/1 -> Gain/1
  SPO2_Context_Risk/1 -> Gain2/1
  TEMP_Context_Risk/1 -> Gain1/1
  Gain/1 -> Sum/1
  Gain2/1 -> Sum/2
  Gain1/1 -> Sum/3
  Sum/1 -> Saturation/1
  Saturation/1 -> Scope/1, Global_Risk_Index/1
  SPO2_Risk_Norm/1 -> Gain3/1
  Gain3/1 -> Sum/4
  HR_Risk_Norm/1 -> Gain5/1
  Gain5/1 -> Sum/5
  Gain4/1 -> Sum/6
  TEMP_Risk_Norm/1 -> Gain4/1

== system Bio_Digital_Twin/Frugal_AI/4.5_Risk_Fusion_Decision_logic/4.5.4_Discrete_Override_Logic ==
  Global_Risk_Index : Inport  OutDataTypeStr=double
  Global_Health_State : Inport  Port=2  OutDataTypeStr=double
  HR_Flag : Inport  Port=3  OutDataTypeStr=double
  TEMP_Flag : Inport  Port=4  OutDataTypeStr=double
  SPO2_Flag : Inport  Port=5  OutDataTypeStr=double
  Constant : Constant  Value=0  OutDataTypeStr=double
  Constant1 : Constant  Value=50  OutDataTypeStr=double
  Constant2 : Constant  Value=100  OutDataTypeStr=double
  Max : MinMax  Function=max  Inputs=3  OutDataTypeStr=double  ZeroCross=off
  Multiport Switch : MultiPortSwitch  DataPortOrder=Zero-based contiguous  zeroidx=on  OutDataTypeStr=double  SaturateOnIntegerOverflow=off  InputSameDT=off
  Relational Operator : RelationalOperator  Operator=>  OutDataTypeStr=boolean  ZeroCross=off  RndMeth=Simplest  InputSameDT=off
  Scope : Scope
      settings: DataLoggingVariableName=ScopeData72  DataLoggingSaveFormat=Array
  Switch : Switch  Criteria=u2 > Threshold  OutDataTypeStr=double  ZeroCross=off  SaturateOnIntegerOverflow=off  InputSameDT=off
  Override_level : Outport  OutDataTypeStr=double  VectorParamsAs1DForOutWhenUnconnected=off
  Out1 : Outport  Port=2  OutDataTypeStr=double  VectorParamsAs1DForOutWhenUnconnected=off
  wires:
  Global_Health_State/1 -> Relational Operator/1
  HR_Flag/1 -> Max/1
  SPO2_Flag/1 -> Max/2
  TEMP_Flag/1 -> Max/3
  Max/1 -> Switch/1, Relational Operator/2
  Relational Operator/1 -> Switch/2
  Global_Risk_Index/1 -> Switch/3
  Constant/1 -> Multiport Switch/1
  Constant1/1 -> Multiport Switch/2
  Constant2/1 -> Multiport Switch/3
  Switch/1 -> Out1/1, Multiport Switch/4
  Multiport Switch/1 -> Override_level/1, Scope/1

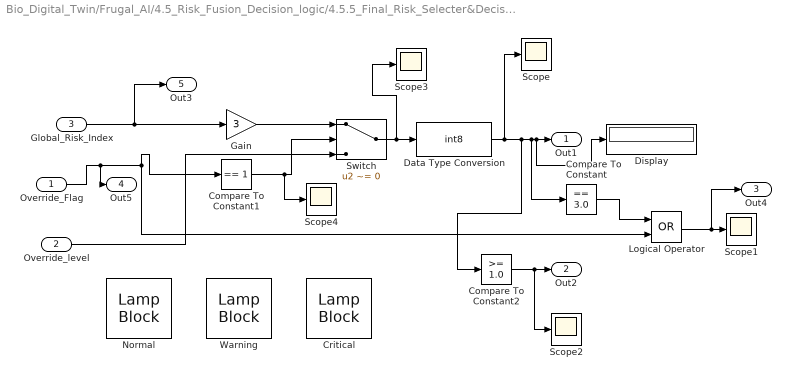
== system Bio_Digital_Twin/Frugal_AI/4.5_Risk_Fusion_Decision_logic/4.5.5_Final_Risk_Selecter&Decision_Output ==
  Override_Flag : Inport  OutDataTypeStr=double
  Override_level : Inport  Port=2  OutDataTypeStr=double
  Global_Risk_Index : Inport  Port=3  OutDataTypeStr=double
  Compare To Constant : simulink/Logic and Bit Operations/Compare To Constant  relop===  const=3.0  OutDataTypeStr=boolean  ZeroCross=off
  Compare To Constant1 : simulink/Logic and Bit Operations/Compare To Constant  relop===  const=1  OutDataTypeStr=boolean  ZeroCross=off
  Compare To Constant2 : simulink/Logic and Bit Operations/Compare To Constant  relop=>=  const=1.0  OutDataTypeStr=boolean  ZeroCross=off
  Critical : LampBlock  LabelPosition=Hide  DefaultColor=[0.0, 0.0, 0.0]
  Data Type Conversion : DataTypeConversion  OutDataTypeStr=int8  SaturateOnIntegerOverflow=off  RndMeth=Floor
  Display : Display
  Gain : Gain  Gain=3  OutDataTypeStr=double
  Logical Operator : Logic  Operator=OR  AllPortsSameDT=off  OutDataTypeStr=boolean
  Normal : LampBlock  LabelPosition=Hide  DefaultColor=[0.0, 0.0, 0.0]
  Scope{,1..4} (5 alike) : Scope
      Scope settings: ActiveDisplayYMinimum=2.03194670986947  ActiveDisplayYMaximum=3.9741968881823517  DataLoggingVariableName=ScopeData73  DataLoggingSaveFormat=Array
      Scope1 settings: ActiveDisplayYMinimum=0.9  ActiveDisplayYMaximum=1.1  DataLoggingVariableName=ScopeData74  DataLoggingSaveFormat=Array
      Scope2 settings: ActiveDisplayYMinimum=0.9  ActiveDisplayYMaximum=1.1  DataLoggingVariableName=ScopeData75  DataLoggingSaveFormat=Array
      Scope3 settings: DataLoggingVariableName=ScopeData79  DataLoggingSaveFormat=Array
      Scope4 settings: ActiveDisplayYMinimum=-1  ActiveDisplayYMaximum=1  DataLoggingVariableName=ScopeData80  DataLoggingSaveFormat=Array
  Switch : Switch  Criteria=u2 ~= 0  OutDataTypeStr=double  ZeroCross=off  SaturateOnIntegerOverflow=off  InputSameDT=off
  Warning : LampBlock  LabelPosition=Hide  DefaultColor=[0.0, 0.0, 0.0]
  Out1 : Outport
  Out2 : Outport  Port=2
  Out4 : Outport  Port=3
  Out5 : Outport  Port=4
  Out3 : Outport  Port=5
  wires:
  Global_Risk_Index/1 -> Out3/1, Gain/1
  Override_Flag/1 -> Out5/1, Compare To Constant1/1, Logical Operator/2
  Gain/1 -> Switch/1
  Compare To Constant1/1 -> Scope4/1, Switch/2
  Override_level/1 -> Switch/3
  Switch/1 -> Scope3/1, Data Type Conversion/1
  Compare To Constant/1 -> Logical Operator/1
  Data Type Conversion/1 -> Scope/1, Compare To Constant2/1, Compare To Constant/1, Display/1, Out1/1
  Logical Operator/1 -> Out4/1, Scope1/1
  Compare To Constant2/1 -> Scope2/1, Out2/1

== system Bio_Digital_Twin/Frugal_AI/4.4_Predective_Health_Estimater/4.4.4_Vital_Fusion_Engine/4.4.4.1_Weighted_Risk_Aggregator ==
  TEMP_Boosted_Risk : Inport
  SPO2_Boosted_Risk : Inport  Port=2
  HR_Boosted_Risk : Inport  Port=3
  Gain : Gain  Gain=[0.35 0.45 0.20]
  Mux : Mux  Inputs=3
  Scope : Scope
      settings: DataLoggingVariableName=ScopeData48  DataLoggingSaveFormat=Array
  R_Weighted : Outport  VectorParamsAs1DForOutWhenUnconnected=off
  wires:
  TEMP_Boosted_Risk/1 -> Mux/1
  SPO2_Boosted_Risk/1 -> Mux/2
  HR_Boosted_Risk/1 -> Mux/3
  Mux/1 -> Gain/1
  Gain/1 -> Scope/1, R_Weighted/1

== system Bio_Digital_Twin/Frugal_AI/4.4_Predective_Health_Estimater/4.4.4_Vital_Fusion_Engine/4.4.4.2_Trend_Reinforcement_Logic ==
  SPO2_Trend_Penality : Inport
  HR_Trend_Penalty : Inport  Port=2
  TEMP_Trend_Penality : Inport  Port=3
  Gain : Gain  Gain=0.6
  Mean : dspstat3/Mean  run=off  InputProcessing=Columns as channels (frame based)  reset_popup=None  directionMode=Each column  dimension=1  roiEnable=off  roiType=Rectangles  roiPortion=Entire ROI  roiOutput=Individual statistics for each ROI  roiFlag=off  roundingMode=Floor  overflowMode=off  outputDataTypeStr=Inherit: Same as accumulator  outputMin=[]  outputMax=[]  outputLastDataTypeStr=Inherit: Same as accumulator
  Mux : Mux  Inputs=3
  Scope : Scope
      settings: DataLoggingVariableName=ScopeData47  DataLoggingSaveFormat=Array
  Trend_Factor : Outport
  wires:
  SPO2_Trend_Penality/1 -> Mux/1
  HR_Trend_Penalty/1 -> Mux/2
  TEMP_Trend_Penality/1 -> Mux/3
  Mux/1 -> Mean/1
  Mean/1 -> Gain/1
  Gain/1 -> Scope/1, Trend_Factor/1

== system Bio_Digital_Twin/Frugal_AI/4.4_Predective_Health_Estimater/4.4.4_Vital_Fusion_Engine/4.4.4.3_Flag_Confidence_Gate ==
  Trend_Factor : Inport
  HR_Flag : Inport  Port=2
  TEMP_Flag : Inport  Port=3
  SPO2_Flag : Inport  Port=4
  Constant : Constant
  Constant1 : Constant  Value=0
  Mux : Mux  Inputs=3
  Relational Operator : RelationalOperator  OutDataTypeStr=boolean  ZeroCross=off  RndMeth=Simplest  InputSameDT=off
  Scope : Scope
      settings: DataLoggingVariableName=ScopeData49  DataLoggingSaveFormat=Array
  Sum : Sum  Inputs=+
  Switch : Switch  Criteria=u2 > Threshold  ZeroCross=off  SaturateOnIntegerOverflow=off  InputSameDT=off
  Risk_Validated : Outport
  wires:
  HR_Flag/1 -> Mux/1
  TEMP_Flag/1 -> Mux/3
  SPO2_Flag/1 -> Mux/2
  Sum/1 -> Relational Operator/2
  Constant/1 -> Relational Operator/1
  Trend_Factor/1 -> Switch/1
  Relational Operator/1 -> Switch/2
  Constant1/1 -> Switch/3
  Switch/1 -> Scope/1, Risk_Validated/1
  Mux/1 -> Sum/1

== system Bio_Digital_Twin/Frugal_AI/4.4_Predective_Health_Estimater/4.4.4_Vital_Fusion_Engine/4.4.4.4_Final_risk_Normalizer ==
  R_Weighted : Inport
  Risk_Validated : Inport  Port=2
  Trend_Factor : Inport  Port=3
  Gain : Gain  Gain=100
  Saturation : Saturate  UpperLimit=100  LowerLimit=0  ZeroCross=off
  Scope : Scope
      settings: DataLoggingVariableName=ScopeData50  DataLoggingSaveFormat=Array
  Sum : Sum  Inputs=|+++
  Vital_Risk_Score : Outport  VectorParamsAs1DForOutWhenUnconnected=off
  wires:
  R_Weighted/1 -> Sum/1
  Trend_Factor/1 -> Sum/2
  Sum/1 -> Gain/1
  Gain/1 -> Saturation/1
  Saturation/1 -> Scope/1, Vital_Risk_Score/1
  Risk_Validated/1 -> Sum/3

== system Bio_Digital_Twin/Frugal_AI/4.4_Predective_Health_Estimater/4.4.4_Vital_Fusion_Engine/4.4.4.5_Decision&Drug_Trigger_Logic ==
  Vital_Risk_Score : Inport
  Constant : Constant  Value=80
  Constant1 : Constant  Value=40
  IS_Danger : RelationalOperator  OutDataTypeStr=boolean  ZeroCross=off  RndMeth=Simplest  InputSameDT=off
  IS_Warning : RelationalOperator  Operator=<=  OutDataTypeStr=boolean  ZeroCross=off  RndMeth=Simplest  InputSameDT=off
  SEV_Danger : Constant  Value=2
  SEV_Normal : Constant  Value=0
  SEV_Warning : Constant
  Scope : Scope
      settings: DataLoggingVariableName=ScopeData51  DataLoggingSaveFormat=Array
  Severity_Select : Switch  Threshold=0.5  ZeroCross=off  SaturateOnIntegerOverflow=off  InputSameDT=off
  Switch : Switch  Threshold=0.5  ZeroCross=off  SaturateOnIntegerOverflow=off  InputSameDT=off
  Risk_Level_Flag : Outport
  wires:
  Vital_Risk_Score/1 -> IS_Warning/1, IS_Danger/1
  Constant/1 -> IS_Danger/2
  Constant1/1 -> IS_Warning/2
  SEV_Warning/1 -> Severity_Select/1
  IS_Warning/1 -> Severity_Select/2
  SEV_Normal/1 -> Severity_Select/3
  SEV_Danger/1 -> Switch/1
  IS_Danger/1 -> Switch/2
  Severity_Select/1 -> Switch/3
  Switch/1 -> Scope/1, Risk_Level_Flag/1

== system Bio_Digital_Twin/Frugal_AI/4.4_Predective_Health_Estimater/4.4.5_Health_State_Encoder/4.4.5.1_Vital_Severity_Normalizer ==
  TEMP_Flag : Inport  OutDataTypeStr=double
  HR_Risk_Score : Inport  Port=2  OutDataTypeStr=double
  Temp_Risk_Output : Inport  Port=3  OutDataTypeStr=double
  SPO2_RIsk_Score : Inport  Port=4  OutDataTypeStr=double
  SPO2_Flag : Inport  Port=5  OutDataTypeStr=double
  HR_Flag : Inport  Port=6  OutDataTypeStr=double
  Gain : Gain  Gain=0.5  OutDataTypeStr=double
  Gain1 : Gain  OutDataTypeStr=double
  Gain2 : Gain  OutDataTypeStr=double
  Saturation : Saturate  UpperLimit=1  LowerLimit=0  ZeroCross=off  OutDataTypeStr=double
  Saturation1 : Saturate  UpperLimit=1  LowerLimit=0  ZeroCross=off  OutDataTypeStr=double
  Saturation2 : Saturate  UpperLimit=1  LowerLimit=0  ZeroCross=off  OutDataTypeStr=double
  Scope : Scope
      settings: DataLoggingVariableName=ScopeData53  DataLoggingSaveFormat=Array
  Scope1 : Scope
      settings: DataLoggingVariableName=ScopeData54  DataLoggingSaveFormat=Array
  Scope2 : Scope
      settings: DataLoggingVariableName=ScopeData55  DataLoggingSaveFormat=Array
  HR_Severity : Outport  OutDataTypeStr=double  VectorParamsAs1DForOutWhenUnconnected=off
  SPO2_Severity : Outport  Port=2  OutDataTypeStr=double  VectorParamsAs1DForOutWhenUnconnected=off
  TEMP_Severity : Outport  Port=3  OutDataTypeStr=double  VectorParamsAs1DForOutWhenUnconnected=off
  wires:
  HR_Flag/1 -> Gain/1
  Gain/1 -> Saturation/1
  SPO2_Flag/1 -> Gain1/1
  Gain1/1 -> Saturation1/1
  Gain2/1 -> Saturation2/1
  TEMP_Flag/1 -> Gain2/1
  Saturation/1 -> Scope/1, HR_Severity/1
  Saturation1/1 -> Scope1/1, SPO2_Severity/1
  Saturation2/1 -> Scope2/1, TEMP_Severity/1

== system Bio_Digital_Twin/Frugal_AI/4.4_Predective_Health_Estimater/4.4.5_Health_State_Encoder/4.4.5.2_Health_Vector_Builder ==
  HR_Severity : Inport  OutDataTypeStr=double
  SPO2_Severity : Inport  Port=2  OutDataTypeStr=double
  TEMP_Severity : Inport  Port=3  OutDataTypeStr=double
  Mux : Mux  Inputs=3
  Scope : Scope
      settings: DataLoggingVariableName=ScopeData52  DataLoggingSaveFormat=Array
  Health_Vector : Outport  VectorParamsAs1DForOutWhenUnconnected=off
  Out1 : Outport  Port=2
  Out2 : Outport  Port=3
  Out3 : Outport  Port=4
  wires:
  HR_Severity/1 -> Out1/1, Mux/1
  TEMP_Severity/1 -> Out3/1, Mux/3
  SPO2_Severity/1 -> Out2/1, Mux/2
  Mux/1 -> Scope/1, Health_Vector/1

== system Bio_Digital_Twin/Frugal_AI/4.4_Predective_Health_Estimater/4.4.5_Health_State_Encoder/4.4.5.3_Weighted_Health_Index_generator ==
  Health_Vector : Inport  OutDataTypeStr=double
  Gain : Gain  Gain=[0.4 0.4 0.2]  OutDataTypeStr=double
  Sum : Sum  Inputs=|+  OutDataTypeStr=double
  Health_Index : Outport  OutDataTypeStr=double
  wires:
  Health_Vector/1 -> Gain/1
  Gain/1 -> Sum/1
  Sum/1 -> Health_Index/1

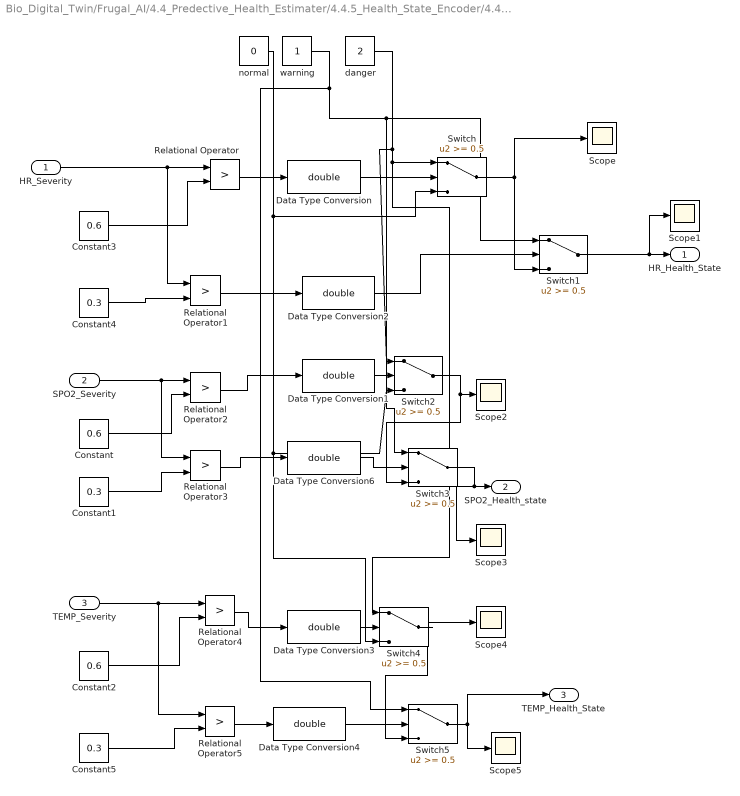
== system Bio_Digital_Twin/Frugal_AI/4.4_Predective_Health_Estimater/4.4.5_Health_State_Encoder/4.4.5.4_Discrete_Health_State_Classifier ==
  HR_Severity : Inport
  SPO2_Severity : Inport  Port=2  OutDataTypeStr=double
  TEMP_Severity : Inport  Port=3  OutDataTypeStr=double
  Constant : Constant  Value=0.6  OutDataTypeStr=double  SampleTime=-1
  Constant1 : Constant  Value=0.3  OutDataTypeStr=double  SampleTime=-1
  Constant2 : Constant  Value=0.6  OutDataTypeStr=double  SampleTime=-1
  Constant3 : Constant  Value=0.6  OutDataTypeStr=double  SampleTime=-1
  Constant4 : Constant  Value=0.3  OutDataTypeStr=double  SampleTime=-1
  Constant5 : Constant  Value=0.3  OutDataTypeStr=double  SampleTime=-1
  Data Type Conversion{,1..4,6} (6 alike) : DataTypeConversion  OutDataTypeStr=double  SaturateOnIntegerOverflow=off  RndMeth=Floor
  Relational Operator{,1..5} (6 alike) : RelationalOperator  Operator=>  OutDataTypeStr=boolean  ZeroCross=off  RndMeth=Simplest  InputSameDT=off
  Scope{,1..5} (6 alike) : Scope
      Scope settings: DataLoggingVariableName=ScopeData56  DataLoggingSaveFormat=Array
      Scope1 settings: DataLoggingVariableName=ScopeData57  DataLoggingSaveFormat=Array
      Scope2 settings: DataLoggingVariableName=ScopeData58  DataLoggingSaveFormat=Array
      Scope3 settings: DataLoggingVariableName=ScopeData59  DataLoggingSaveFormat=Array
      Scope4 settings: DataLoggingVariableName=ScopeData60  DataLoggingSaveFormat=Array
      Scope5 settings: DataLoggingVariableName=ScopeData61  DataLoggingSaveFormat=Array
  Switch{,1..5} (6 alike) : Switch  Threshold=0.5  OutDataTypeStr=double  ZeroCross=off  SaturateOnIntegerOverflow=off  InputSameDT=off
  danger : Constant  Value=2  OutDataTypeStr=double  SampleTime=-1
  normal : Constant  Value=0  OutDataTypeStr=double  SampleTime=-1
  warning : Constant  OutDataTypeStr=double  SampleTime=-1
  HR_Health_State : Outport  OutDataTypeStr=double  VectorParamsAs1DForOutWhenUnconnected=off
  SPO2_Health_state : Outport  Port=2  OutDataTypeStr=double
  TEMP_Health_State : Outport  Port=3  OutDataTypeStr=double
  wires:
  HR_Severity/1 -> Relational Operator1/1, Relational Operator/1
  Constant3/1 -> Relational Operator/2
  Constant4/1 -> Relational Operator1/2
  danger/1 -> Switch4/1, Switch/1, Switch2/1
  Relational Operator/1 -> Data Type Conversion/1
  normal/1 -> Switch4/3, Switch2/3, Switch/3
  warning/1 -> Switch5/1, Switch3/1, Switch1/1
  Relational Operator1/1 -> Data Type Conversion2/1
  Switch/1 -> Switch1/3, Scope/1
  Switch1/1 -> Scope1/1, HR_Health_State/1
  SPO2_Severity/1 -> Relational Operator3/1, Relational Operator2/1
  Constant/1 -> Relational Operator2/2
  Constant1/1 -> Relational Operator3/2
  Relational Operator2/1 -> Data Type Conversion1/1
  Relational Operator3/1 -> Data Type Conversion6/1
  Switch2/1 -> Switch3/3, Scope2/1
  Switch3/1 -> Scope3/1, SPO2_Health_state/1
  Switch4/1 -> Switch5/3, Scope4/1
  Switch5/1 -> TEMP_Health_State/1, Scope5/1
  Relational Operator4/1 -> Data Type Conversion3/1
  Relational Operator5/1 -> Data Type Conversion4/1
  Constant5/1 -> Relational Operator5/2
  Constant2/1 -> Relational Operator4/2
  TEMP_Severity/1 -> Relational Operator5/1, Relational Operator4/1
  Data Type Conversion/1 -> Switch/2
  Data Type Conversion2/1 -> Switch1/2
  Data Type Conversion1/1 -> Switch2/2
  Data Type Conversion4/1 -> Switch5/2
  Data Type Conversion3/1 -> Switch4/2
  Data Type Conversion6/1 -> Switch3/2

== system Bio_Digital_Twin/Frugal_AI/4.4_Predective_Health_Estimater/4.4.5_Health_State_Encoder/4.4.5.5_Final_Decision ==
  Health_Index : Inport  OutDataTypeStr=double
  HR_Health_State : Inport  Port=2  OutDataTypeStr=double
  SPO2_Health_state : Inport  Port=3  OutDataTypeStr=double
  TEMP_Health_State : Inport  Port=4  OutDataTypeStr=double
  Max : MinMax  Function=max  OutDataTypeStr=double
  Mux : Mux
  Scope : Scope
      settings: ActiveDisplayYMinimum=-0.12499999999999997  ActiveDisplayYMaximum=1.125  DataLoggingVariableName=ScopeData62  DataLoggingSaveFormat=Array
  Scope1 : Scope
      settings: ActiveDisplayYMinimum=-0.37211602393617016  ActiveDisplayYMaximum=1.0060089760638298  DataLoggingVariableName=ScopeData63  DataLoggingSaveFormat=Array
  Global_Health_State : Outport  OutDataTypeStr=double
  wires:
  SPO2_Health_state/1 -> Mux/2
  HR_Health_State/1 -> Mux/1
  TEMP_Health_State/1 -> Mux/3
  Mux/1 -> Scope1/1, Max/1
  Max/1 -> Scope/1, Global_Health_State/1
  Health_Index/1 -> Mux/4

== matlab function Bio_Digital_Twin/Drug_Physiology _Intraction Twin/3.2_Pharmacokinetics/MATLAB Function ==
  data: dose input; C_plasma output; patient_factor input
function C_plasma = pharmacokinetics(dose, patient_factor)
% Pharmacokinetics model (exam-safe, deterministic)
% dose           : drug dose (0–10)
% patient_factor : metabolism sensitivity (0.8–1.2)

% --- Drug parameters ---
bioavailability = 0.85;     % fraction absorbed
clearance_rate  = 0.25;     % clearance constant
half_life       = 4;        % hours (normalized time)

% --- Absorbed dose ---
absorbed = dose * bioavailability;

% --- Clearance & decay ---
C_plasma = absorbed .* exp(-clearance_rate .* patient_factor);

% --- Safety saturation ---
if C_plasma > 1
    C_plasma = 1;
elseif C_plasma < 0
    C_plasma = 0;
end
end
